simulink model "non_linear_simulation_2017a"  (R2017a)
settings: Solver=ode4  StartTime=0.0  StopTime=inf  FixedStep=0.01  RelTol=1e-3
libraries: realtime_pacer_lib x1, simulink x1
settings Model: Creator=engen  LastModifiedBy=eirik.engen
settings DataIOCC: ReturnWorkspaceOutputs=on
settings SFSimCC: SimUseLocalCustomCode=on
settings RTWCC: RTWUseLocalCustomCode=on

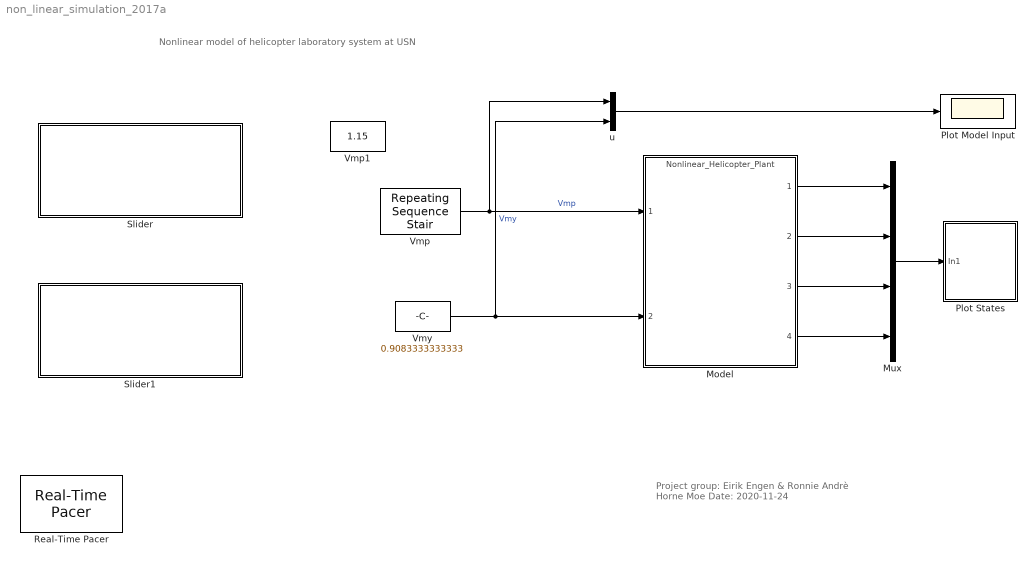
== system non_linear_simulation_2017a ==
  note: Project group:
      | Eirik Engen & Ronnie Andrè Horne Moe
      | Date: 2020-11-24
  note: Nonlinear model of helicopter laboratory system at USN
  Model : ModelReference  ModelNameDialog=Nonlinear_Helicopter_Plant.slxp  ModelReferenceVersion=1.53  CopyOfModelProtected=on
  Mux : Mux
  Plot Model Input : Scope
  Plot States : Subsystem
  Real-Time Pacer : realtime_pacer_lib/Real-Time Pacer  simTimePerRealTime=1
  Slider : Subsystem  DialogController=hmiCreateDDGDialog  IsWebBlock=on  mask(MWDashboardBlock){webBlockId=b02f8cde-b384-4595-a1f7-557cc2f8eea0, webBlockType=slider, ShowInLibBrowser=on, ShowInitialText=on, HMISrcModelName=non_linear_simulation_2017a}
      mask prompts: webBlockId "WebBlock Id"; webBlockType "WebBlock Type"; HMISrcModelName "Source Model"
      mask help: Set value to tune parameters or variables.
      mask Help: helpview([docroot '/mapfiles/simulink.map'], 'hmi_slider')
      mask Display:
      | if strcmp(get_param(bdroot(gcb),'BlockDiagramType'),'library')
      |  image([(matlabroot) '/toolbox/simulink/hmi/icons/Slider.png'])
      | end
  Slider1 : Subsystem  DialogController=hmiCreateDDGDialog  IsWebBlock=on  mask(MWDashboardBlock){webBlockId=814737d5-0d92-4344-bbdd-3ac21f161371, webBlockType=slider, ShowInLibBrowser=on, ShowInitialText=on, HMISrcModelName=non_linear_simulation_2017a}
      mask prompts: webBlockId "WebBlock Id"; webBlockType "WebBlock Type"; HMISrcModelName "Source Model"
      mask help: Set value to tune parameters or variables.
      mask Help: helpview([docroot '/mapfiles/simulink.map'], 'hmi_slider')
      mask Display:
      | if strcmp(get_param(bdroot(gcb),'BlockDiagramType'),'library')
      |  image([(matlabroot) '/toolbox/simulink/hmi/icons/Slider.png'])
      | end
  Vmp : simulink/Sources/Repeating Sequence Stair  OutValues=[1.25 1.2 1.15 1.1 1.2 1.3].'  tsamp=15  OutMin=[]  OutMax=[]  OutDataTypeStr=double  OutputDataTypeScalingMode=double  OutDataType=fixdt(0,8)  ConRadixGroup=Best Precision: Vector-wise  OutScaling=2^-12
  Vmp1 : Constant  Value=1.15  SampleTime=-1
  Vmy : Constant  Value=0.9083333333333  SampleTime=-1
  u : Mux  Inputs=2
  wires:
  Mux/1 -> Plot States/1(In1)
  u/1 -> Plot Model Input/1
  Model/1 -> Mux/1
  Model/2 -> Mux/2
  Model/3 -> Mux/3
  Model/4 -> Mux/4
  Vmp/1 -> u/1, Model/1  "Vmp"
  Vmy/1 -> u/2, Model/2  "Vmy"

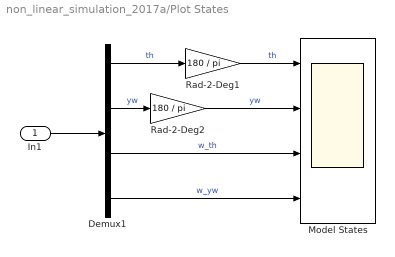
== system non_linear_simulation_2017a/Plot States ==
  In1 : Inport
  Demux1 : Demux
  Model States : Scope  NumInputPorts=4
  Rad-2-Deg1 : Gain  Gain=180 / pi
  Rad-2-Deg2 : Gain  Gain=180 / pi
  wires:
  Demux1/2 -> Rad-2-Deg2/1  "yw"
  Demux1/3 -> Model States/3  "w_th"
  Demux1/1 -> Rad-2-Deg1/1  "th"
  Demux1/4 -> Model States/4  "w_yw"
  In1/1 -> Demux1/1
  Rad-2-Deg1/1 -> Model States/1  "th"
  Rad-2-Deg2/1 -> Model States/2  "yw"

== system non_linear_simulation_2017a/Slider ==

== system non_linear_simulation_2017a/Slider1 ==
